simulink model "proiectbun"  (R2015a)
settings: Solver=ode23  StartTime=0.0  StopTime=20000.0  FixedStep=1  RelTol=1e-3
settings Model: Creator=Laptop Horia  LastModifiedBy=Horia

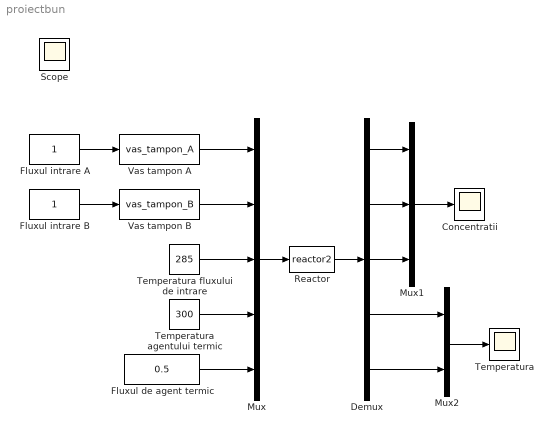
== system proiectbun ==
  Concentratii : Scope
      settings: YMin=0.8  YMax=2.1  MaxDataPoints=500000
  Demux : Demux  Outputs=5
  Fluxul de agent termic : Constant  Value=0.5
  Fluxul intrare A : Constant
  Fluxul intrare B : Constant
  Mux : Mux  Inputs=5
  Mux1 : Mux  Inputs=3
  Mux2 : Mux  Inputs=2
  Reactor : S-Function  FunctionName=reactor2
  "Temperatura " : Scope
      settings: YMin=262.5  YMax=300  SaveName=ScopeData2  MaxDataPoints=500000
  Temperatura agentului termic : Constant  Value=300
  Temperatura fluxului de intrare : Constant  Value=285
  Vas tampon A : S-Function  FunctionName=vas_tampon_A
  Vas tampon B : S-Function  FunctionName=vas_tampon_B
  Scope : Scope
      settings: SaveName=ScopeData3
  wires:
  Mux/1 -> Reactor/1
  Reactor/1 -> Demux/1
  Demux/1 -> Mux1/1
  Demux/2 -> Mux1/2
  Demux/3 -> Mux1/3
  Demux/4 -> Mux2/1
  Temperatura fluxului de intrare/1 -> Mux/3
  Temperatura agentului termic/1 -> Mux/4
  Fluxul de agent termic/1 -> Mux/5
  Demux/5 -> Mux2/2
  Mux2/1 -> "Temperatura "/1
  Mux1/1 -> Concentratii/1
  Fluxul intrare A/1 -> Vas tampon A/1
  Fluxul intrare B/1 -> Vas tampon B/1
  Vas tampon A/1 -> Mux/1
  Vas tampon B/1 -> Mux/2
